simulink library "Displays_Lib"  (Simulink 6.6)
PostLoadFcn:
  | ,try, rti_mdl_postloadfcn(bdroot, 'UpdateModel', 260, 'rti1005'); catch, disp(lasterr); end,
undefined symbols (not defined in the file or in its folder): Timestep
libraries: Displays_Lib x5, udpbs x4, simulink x1
settings Model: Creator=W.J.Leath  LastModifiedBy=cbuttril  ExtModeAutoUpdateStatusClock=off

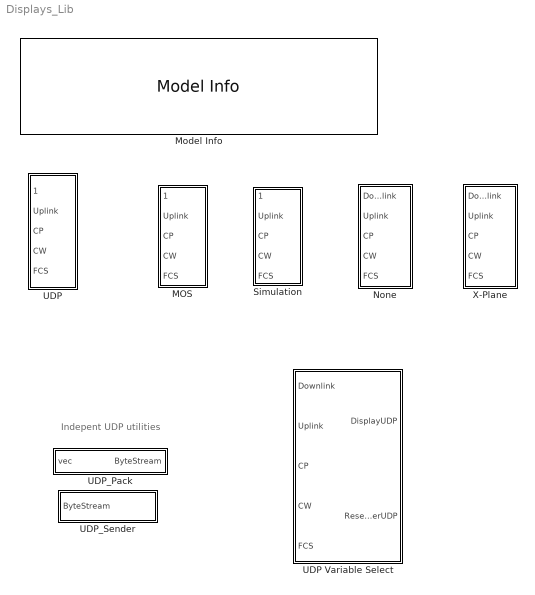
== system Displays_Lib ==
  note: Indepent UDP utilities
  MOS : Subsystem
  Model Info : simulink/Model-Wide Utilities/Model Info  SystemSampleTime=-1  InitialBlockCM=None  BlockCM=None  Frame=on  DisplayStringWithTags=|  HorizontalTextAlignment=Center  LeftAlignmentValue=0.5  SourceBlockDiagram=Displays_Lib  TagMaxNumber=20
      | Developed using Matlab Release 2007a
      | 
      | SVN:%<ModelVersion>
      | Modified: %<ModifiedDate>
  None : Subsystem
  Simulation : Subsystem
  UDP : Subsystem  BlockChoice=MOS
      settings: TemplateBlock=self  MemberBlocks=MOS,None,Simulation,X-Plane
  UDP Variable Select : Subsystem
  UDP_Pack : Subsystem  mask(UDPPacker){DataType=double, EndianListNdx=Little Endian (Intel)}
      mask prompts: DataType "Input datatype"; EndianListNdx "Native Byte Order"
      mask help: Takes vectors of doubles or uint32s and forms a packed bytestream suitable for sending via UDP.
      mask init:
      | IsBigEndian=boolean(EndianListNdx-1);
      | switch DataType
      |     case 'uint32'
      |         vbytes = 4;
      |     case 'double'
      |         vbytes = 8;
      | end
      mask StyleString: popup(uint32|double),popup(Little Endian (Intel)|Big Endian (dSpace))
      mask Display:
      | port_label('input',1,DataType)
      | port_label('output',1,'ByteStream')
  UDP_Sender : Subsystem  mask(UDP_Send){UDP_Port=5001}
      mask prompts: UDP_Port "UDP Port to Send Message to"
      mask help: Sends a uint8 bytesteam to the specified UDP port. Must be able to open a different port on local machine to estabilish the socket. By convention the local socket is opened one port below the destination port. For example, to send a message to port 5001, this block must be able to open a socket on port 5000 on the local machine.
  X-Plane : Subsystem

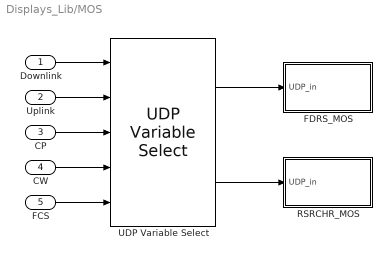
== system Displays_Lib/MOS ==
  Downlink : Inport
  Uplink : Inport  Port=2
  CP : Inport  Port=3
  CW : Inport  Port=4
  FCS : Inport  Port=5
  FDRS_MOS : Subsystem
  RSRCHR_MOS : Subsystem
  UDP Variable Select : Displays_Lib/UDP Variable Select  SystemSampleTime=-1
      link override UDP_Pack: EndianListNdx=Big Endian (dSpace)
      link override UDP_Pack0: EndianListNdx=Big Endian (dSpace)
      link override UDP_Pack1: EndianListNdx=Big Endian (dSpace)
      link override UDP_Pack2: EndianListNdx=Big Endian (dSpace)
      link override UDP_Pack3: EndianListNdx=Big Endian (dSpace)
  wires:
  Downlink/1 -> UDP Variable Select/1
  Uplink/1 -> UDP Variable Select/2
  CP/1 -> UDP Variable Select/3
  FCS/1 -> UDP Variable Select/5
  CW/1 -> UDP Variable Select/4
  UDP Variable Select/1 -> FDRS_MOS/1(UDP_in)
  UDP Variable Select/2 -> RSRCHR_MOS/1(UDP_in)

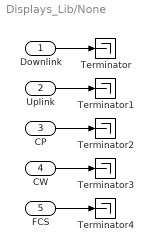
== system Displays_Lib/None ==
  Downlink : Inport
  Uplink : Inport  Port=2
  CP : Inport  Port=3
  CW : Inport  Port=4
  FCS : Inport  Port=5
  Terminator{,1..4} (5 alike) : Terminator
  wires:
  Downlink/1 -> Terminator/1
  Uplink/1 -> Terminator1/1
  CP/1 -> Terminator2/1
  CW/1 -> Terminator3/1
  FCS/1 -> Terminator4/1

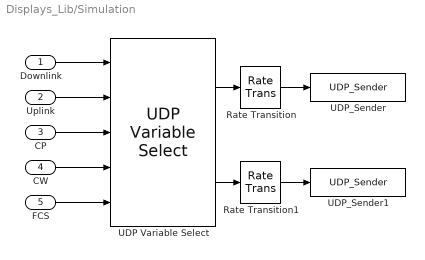
== system Displays_Lib/Simulation ==
  Downlink : Inport
  Uplink : Inport  Port=2
  CP : Inport  Port=3
  CW : Inport  Port=4
  FCS : Inport  Port=5
  Rate Transition : RateTransition  Deterministic=off  OutPortSampleTime=Timestep*4
  Rate Transition1 : RateTransition  Deterministic=off  OutPortSampleTime=Timestep*4
  UDP Variable Select : Displays_Lib/UDP Variable Select  SystemSampleTime=-1
  UDP_Sender : Displays_Lib/UDP_Sender  SystemSampleTime=-1  UDP_Port=5500
  UDP_Sender1 : Displays_Lib/UDP_Sender  SystemSampleTime=-1  UDP_Port=5700
  wires:
  Downlink/1 -> UDP Variable Select/1
  Uplink/1 -> UDP Variable Select/2
  CP/1 -> UDP Variable Select/3
  FCS/1 -> UDP Variable Select/5
  CW/1 -> UDP Variable Select/4
  UDP Variable Select/1 -> Rate Transition/1
  UDP Variable Select/2 -> Rate Transition1/1
  Rate Transition/1 -> UDP_Sender/1
  Rate Transition1/1 -> UDP_Sender1/1

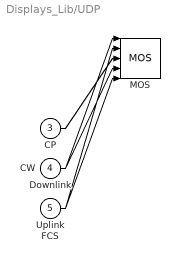
== system Displays_Lib/UDP ==
  Downlink : Inport
  Uplink : Inport  Port=2
  CP : Inport  Port=3
  CW : Inport  Port=4
  FCS : Inport  Port=5
  MOS : Displays_Lib/MOS  SystemSampleTime=-1
  wires:
  Downlink/1 -> MOS/1
  Uplink/1 -> MOS/2
  CP/1 -> MOS/3
  CW/1 -> MOS/4
  FCS/1 -> MOS/5

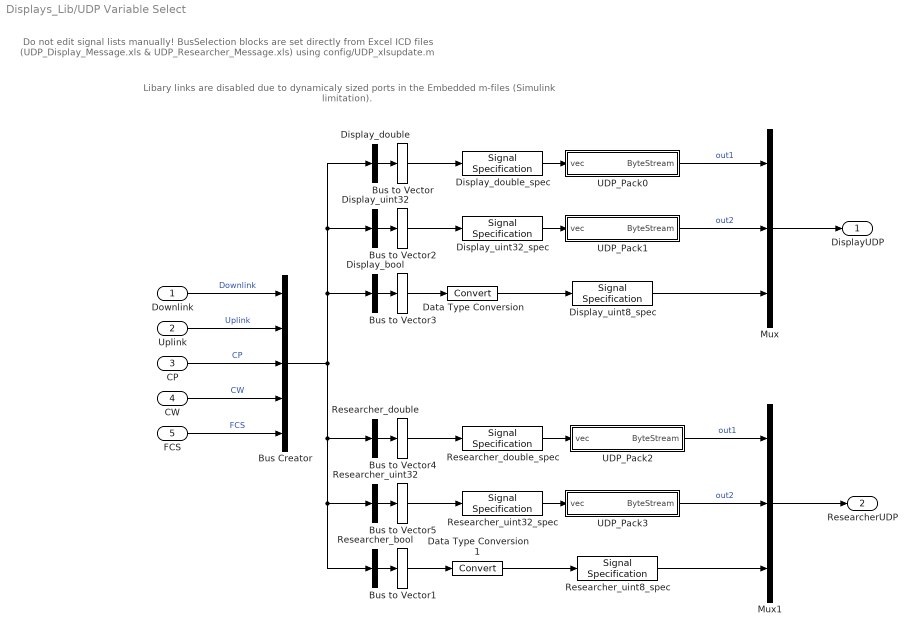
== system Displays_Lib/UDP Variable Select ==
  note: Libary links are disabled due to dynamicaly sized ports
      | in the Embedded m-files (Simulink limitation).
  note: Do not edit signal lists manually!  BusSelection blocks are set directly from Excel ICD files
      | (UDP_Display_Message.xls & UDP_Researcher_Message.xls) using config/UDP_xlsupdate.m
  Downlink : Inport
  Uplink : Inport  Port=2
  CP : Inport  Port=3
  CW : Inport  Port=4
  FCS : Inport  Port=5
  Bus Creator : BusCreator  Inputs=5
  Bus to Vector{,1..5} (6 alike) : BusToVector
  Data Type Conversion : DataTypeConversion  OutDataTypeMode=uint8
  Data Type Conversion1 : DataTypeConversion  OutDataTypeMode=uint8
  Display_bool : BusSelector  OutputSignals=FCS.RPraw.FTE_mark,FCS.RPraw.TD_mark,FCS.RPraw.ENG_mark,FCS.RPraw.RES_mark,FCS.SPInput.gear_cmd,FCS.SPInput.handoff_switch,FCS.RPInput.Fuel_Intg,CW.LinkInop  OutputAsBus=on
  Display_double : BusSelector  OutputSignals=CP.AirData.vc,CP.AirData.vt,CP.CGVanesAcc.gwest,CP.Display.cg_mac,CP.Display.vstall_est_disp,CP.Display.vc_disp,CP.Display.alpha_disp,CP.Display.beta_disp,CP.Display.baro_alt,CP.Display.nz_disp,CP.Display.vv_fpm_disp,CP.Display.mag_heading_disp,CP.Display.alt_gps_disp,CP.Display.BUSMON1_disp,CP.Display.BUSMON2_disp,CP.Display.BUSMON3_disp,CP.Display.BUSMON4_disp,CP.Display.CPTV_disp,CP.Display.BAROV_disp,CP.Display.MAG3V_disp,CP.Display.RSS_disp,CP.Display.DL_RSS_disp,CP.Engine_Fuel.fuel_rem,CP.Engine_Fuel.fuel_flow_l,CP.Engine_Fuel.fuel_flow_r,CP.Engine_Fuel.fuel_used,CP.Engine_Fuel.time_rem,CP.Engine_Fuel.rpm_left,CP.Engine_Fuel.rpm_right,CP.Engine_Fuel.rpml_ATcmd,CP.Engine_Fuel.rpmr_ATcmd,CP.Engine_Fuel.rpml_RPcmd,CP.Engine_Fuel.rpmr_RPcmd,CP.Engine_Fuel.rpml_SPcmd,CP.Engine_Fuel.rpmr_SPcmd,CP.Nav.vcdot,CP.Nav.vgnav,CP.Nav.windspd,CP.Nav.winddir,CP.Nav.gammav,CP.Nav.gndtrack,CP.Surfaces.RPele_cmd,CP.Surfaces.aildiff,CP.Surfaces.elevave,CP.Surfaces.rudave,CP.CP_constants.altimeter_setting,CP.Offset_Landing.baro_alt_HUD,CP.Offset_Landing.mag_heading_disp_HUD,CP.Offset_Landing.gndtrack_HUD,CP.Offset_Landing.psideg_HUD,CP.Offset_Landing.latdeg_HUD,CP.Offset_Landing.londeg_HUD,Downlink.ADC.EGTR,Downlink.ADC.EGTL,Downlink.ADC.SSCS,Downlink.ADC.PSL,Downlink.ADC.PDL,Downlink.ADC.PSR,Downlink.ADC.PDR,Downlink.ADC.AILL,Downlink.ADC.AILR,Downlink.ADC.ELLOB,Downlink.ADC.ELLIB,Downlink.ADC.ELROB,Downlink.ADC.ELRIB,Downlink.ADC.RUDU,Downlink.ADC.RUDL,Downlink.ADC.XACCEL,Downlink.ADC.YACCEL,Downlink.ADC.ZACCEL,Downlink.ADC.XGYRO,Downlink.ADC.YGYRO,Downlink.ADC.ZGYRO,Downlink.ADC.TEMPAMB,Downlink.Health.PacketErrorIndPort0,Downlink.Health.PacketErrorIndPort1,Downlink.Health.PacketErrorIndPort2,Downlink.Health.PacketErrorIndPort3,Downlink.MIDG.MSG_10.TimeStamp,Downlink.MIDG.MSG_10.pdeg,Downlink.MIDG.MSG_10.qdeg,Downlink.MIDG.MSG_10.rdeg,Downlink.MIDG.MSG_10.nxbody,Downlink.MIDG.MSG_10.nybody,Downlink.MIDG.MSG_10.nzbody,Downlink.MIDG.MSG_10.phideg,Downlink.MIDG.MSG_10.thetadeg,Downlink.MIDG.MSG_10.psideg,Downlink.MIDG.MSG_12.LAT_NAV,Downlink.MIDG.MSG_12.LON_NAV,Downlink.MIDG.MSG_1.MIDG_mode,FCS.AT.spd_cmd,FCS.Mode2.beta_cmd,FCS.Mode2.alpha_trim_cmd,FCS.Mode2.alpha_cmd,FCS.RPInput.throttle_L,FCS.RPInput.throttle_R,FCS.RPInput.lon_stk,FCS.RPInput.lat_stk,FCS.RPInput.pedal,FCS.RPInput.hat_lon,FCS.RPInput.hat_lat,FCS.RPInput.flap,FCS.RPInput.spd_brake,FCS.RPInput.Alpha_select,FCS.RPInput.Beta_select,FCS.RPInput.DynPress_select,FCS.RPInput.StatPress_select,FCS.Uplink_cmds.ELLOBC,FCS.Uplink_cmds.ELLIBC,FCS.Uplink_cmds.ELROBC,FCS.Uplink_cmds.ELRIBC,FCS.Uplink_cmds.AILLC,FCS.Uplink_cmds.SPLLOBC,FCS.Uplink_cmds.SPLLIBC,FCS.Uplink_cmds.SPLRIBC,FCS.Uplink_cmds.SPLROBC,FCS.Uplink_cmds.AILRC,FCS.Uplink_cmds.RUDUPC,FCS.Uplink_cmds.RUDLOC,FCS.Uplink_cmds.FLAPLOC,FCS.Uplink_cmds.FLAPLIC,FCS.Uplink_cmds.FLAPRIC,FCS.Uplink_cmds.FLAPROC,FCS.Uplink_cmds.GEARC,FCS.SPInput.throttle_cmd,FCS.SPInput.ail_cmd,FCS.SPInput.ele_cmd,FCS.SPInput.rud_cmd,FCS.SPInput.flap_cmd  OutputAsBus=on
  Display_double_spec : SignalSpecification  Dimensions=130  DataType=double
  Display_uint32 : BusSelector  OutputSignals=CW.warning_word,CW.caution_word,CW.advisory_word,FCS.FCS_Engage,FCS.FCS_Arm,FCS.Wavetrain.WT_status.WT_profile,FCS.Mode3.rFCL_select,FCS.MTF.MTF_profile,CW.StallTone  OutputAsBus=on
  Display_uint32_spec : SignalSpecification  Dimensions=9  DataType=uint32
  Display_uint8_spec : SignalSpecification  Dimensions=8  DataType=uint8
  Mux : Mux  Inputs=3
  Mux1 : Mux  Inputs=3
  Researcher_bool : BusSelector  OutputSignals=FCS.RPraw.gear  OutputAsBus=on
  Researcher_double : BusSelector  OutputSignals=Downlink.ADC.ALPHAVL,Downlink.ADC.BETAVL,Downlink.ADC.ALPHAVR,Downlink.ADC.BETAVR,Downlink.ADC.PSL,Downlink.ADC.PDL,Downlink.ADC.PSR,Downlink.ADC.PDR,Downlink.ADC.XACCEL,Downlink.ADC.YACCEL,Downlink.ADC.ZACCEL,Downlink.ADC.XGYRO,Downlink.ADC.YGYRO,Downlink.ADC.ZGYRO,Downlink.ADC.XMAG,Downlink.ADC.YMAG,Downlink.ADC.ZMAG,Downlink.ADC.XGYROT,Downlink.ADC.AILL,Downlink.ADC.AILR,Downlink.ADC.ELLOB,Downlink.ADC.ELLIB,Downlink.ADC.ELROB,Downlink.ADC.ELRIB,Downlink.ADC.RUDU,Downlink.ADC.RUDL,Downlink.ADC.FLAPLOB,Downlink.ADC.FLAPLIB,Downlink.ADC.FLAPRIB,Downlink.ADC.FLAPROB,Downlink.ADC.TEMPAMB,Downlink.ADC.RPML,Downlink.ADC.RPMR,Downlink.MIDG.MSG_10.TimeStamp,Downlink.MIDG.MSG_10.pdeg,Downlink.MIDG.MSG_10.qdeg,Downlink.MIDG.MSG_10.rdeg,Downlink.MIDG.MSG_10.nxbody,Downlink.MIDG.MSG_10.nybody,Downlink.MIDG.MSG_10.nzbody,Downlink.MIDG.MSG_10.phideg,Downlink.MIDG.MSG_10.thetadeg,Downlink.MIDG.MSG_10.psideg,Downlink.MIDG.MSG_10.QW,Downlink.MIDG.MSG_10.QX,Downlink.MIDG.MSG_10.QY,Downlink.MIDG.MSG_10.QZ,Downlink.MIDG.MSG_12.LAT_NAV,Downlink.MIDG.MSG_12.LON_NAV,Downlink.MIDG.MSG_12.HELIP_NAV,Downlink.MIDG.MSG_12.VEE_NAV,Downlink.MIDG.MSG_12.VN_NAV,Downlink.MIDG.MSG_12.VH_NAV,Uplink.AILLC,Uplink.AILRC,Uplink.ELLOBC,Uplink.ELLIBC,Uplink.ELROBC,Uplink.ELRIBC,Uplink.RUDUPC,Uplink.RUDLOC,Uplink.FLAPLIC,Uplink.FLAPLOC,Uplink.FLAPRIC,Uplink.FLAPROC,Uplink.THROTLC,Uplink.THROTRC,Uplink.GEARC,Uplink.SPLLIBC,Uplink.SPLLOBC,Uplink.SPLRIBC,Uplink.SPLROBC,CP.CGVanesAcc.gwest,CP.CGVanesAcc.cgx,CP.CGVanesAcc.cgy,CP.CGVanesAcc.cgz,CP.CGVanesAcc.ixx,CP.CGVanesAcc.iyy,CP.CGVanesAcc.izz,CP.CGVanesAcc.ixz,CP.CGVanesAcc.MIDG_nxcorr,CP.CGVanesAcc.MIDG_nycorr,CP.CGVanesAcc.MIDG_nzcorr,CP.CGVanesAcc.nxcorr,CP.CGVanesAcc.nycorr,CP.CGVanesAcc.nzcorr,CP.CGVanesAcc.alpha_l,CP.CGVanesAcc.beta_l,CP.CGVanesAcc.alpha_r,CP.CGVanesAcc.beta_r,CP.AirData.vt,CP.AirData.hpic,CP.Nav.windspd,CP.Nav.winddir,CP.Engine_Fuel.fuel_used,CP.Engine_Fuel.rpm_left,CP.Engine_Fuel.rpm_right,CP.Surfaces.aildiff,CP.Surfaces.elevave,CP.Surfaces.rudave,FCS.RPraw.throttle_L,FCS.RPraw.throttle_R,FCS.RPraw.lon_stk,FCS.RPraw.lat_stk,FCS.RPraw.pedal,FCS.RPraw.hat_lon,FCS.RPraw.hat_lat,FCS.RPraw.flap,FCS.RPraw.spd_brake,FCS.AT.spd_cmd,FCS.Mode2.beta_cmd,FCS.Mode2.alpha_trim_cmd,FCS.Mode2.alpha_cmd,FCS.Wavetrain.WT_cmds.dAILLC,FCS.Wavetrain.WT_cmds.dAILRC,FCS.Wavetrain.WT_cmds.dELLOBC,FCS.Wavetrain.WT_cmds.dELLIBC,FCS.Wavetrain.WT_cmds.dELROBC,FCS.Wavetrain.WT_cmds.dELRIBC,FCS.Wavetrain.WT_cmds.dRUDUPC,FCS.Wavetrain.WT_cmds.dRUDLOC,FCS.Wavetrain.WT_cmds.dFLAPLIC,FCS.Wavetrain.WT_cmds.dFLAPLOC,FCS.Wavetrain.WT_cmds.dFLAPRIC,FCS.Wavetrain.WT_cmds.dFLAPROC,FCS.Wavetrain.WT_cmds.dTHROTLC,FCS.Wavetrain.WT_cmds.dTHROTRC,FCS.Wavetrain.WT_cmds.dSPLLIBC,FCS.Wavetrain.WT_cmds.dSPLLOBC,FCS.Wavetrain.WT_cmds.dSPLRIBC,FCS.Wavetrain.WT_cmds.dSPLROBC,FCS.Mode3.UserData.UserData1,FCS.Mode3.UserData.UserData2,FCS.Mode3.UserData.UserData3,FCS.Mode3.UserData.UserData4,FCS.Mode3.UserData.UserData5,FCS.Mode3.UserData.UserData6,FCS.Mode3.UserData.UserData7,FCS.Mode3.UserData.UserData8,FCS.Mode3.UserData.UserData9,FCS.Mode3.UserData.UserData10,FCS.Mode3.UserData.UserData11,FCS.Mode3.UserData.UserData12,FCS.Mode3.UserData.UserData13,FCS.Mode3.UserData.UserData14,FCS.Mode3.UserData.UserData15,FCS.Mode3.UserData.UserData16,FCS.Mode3.UserData.UserData17,FCS.Mode3.UserData.UserData18,FCS.Mode3.UserData.UserData19,FCS.Mode3.UserData.UserData20,FCS.Mode3.UserData.UserData21,FCS.Mode3.UserData.UserData22,FCS.Mode3.UserData.UserData23,FCS.Mode3.UserData.UserData24,FCS.Mode3.UserData.UserData25,FCS.Mode3.UserData.UserData26,FCS.Mode3.UserData.UserData27,FCS.Mode3.UserData.UserData28,FCS.Mode3.UserData.UserData29,FCS.Mode3.UserData.UserData30  OutputAsBus=on
  Researcher_double_spec : SignalSpecification  Dimensions=161  DataType=double
  Researcher_uint32 : BusSelector  OutputSignals=FCS.FCS_Engage,FCS.FCS_Arm,FCS.Mode3.rFCL_select,FCS.MTF.MTF_profile,FCS.Wavetrain.WT_status.WT_profile  OutputAsBus=on
  Researcher_uint32_spec : SignalSpecification  Dimensions=5  DataType=uint32
  Researcher_uint8_spec : SignalSpecification  Dimensions=1  DataType=uint8
  UDP_Pack0 : Subsystem  AncestorBlock=Displays_Lib/UDP_Pack  mask(UDPPacker){DataType=double, EndianListNdx=Little Endian (Intel)}
      mask prompts: DataType "Input datatype"; EndianListNdx "Native Byte Order"
      mask help: Takes vectors of doubles or uint32s and forms a packed bytestream suitable for sending via UDP.
      mask init:
      | IsBigEndian=boolean(EndianListNdx-1);
      | switch DataType
      |     case 'uint32'
      |         vbytes = 4;
      |     case 'double'
      |         vbytes = 8;
      | end
      mask StyleString: popup(uint32|double),popup(Little Endian (Intel)|Big Endian (dSpace))
      mask Display:
      | port_label('input',1,DataType)
      | port_label('output',1,'ByteStream')
  UDP_Pack1 : Subsystem  AncestorBlock=Displays_Lib/UDP_Pack  mask(UDPPacker){DataType=uint32, EndianListNdx=Little Endian (Intel)}
      mask prompts: DataType "Input datatype"; EndianListNdx "Native Byte Order"
      mask help: Takes vectors of doubles or uint32s and forms a packed bytestream suitable for sending via UDP.
      mask init:
      | IsBigEndian=boolean(EndianListNdx-1);
      | switch DataType
      |     case 'uint32'
      |         vbytes = 4;
      |     case 'double'
      |         vbytes = 8;
      | end
      mask StyleString: popup(uint32|double),popup(Little Endian (Intel)|Big Endian (dSpace))
      mask Display:
      | port_label('input',1,DataType)
      | port_label('output',1,'ByteStream')
  UDP_Pack2 : Subsystem  AncestorBlock=Displays_Lib/UDP_Pack  mask(UDPPacker){DataType=double, EndianListNdx=Little Endian (Intel)}
      mask prompts: DataType "Input datatype"; EndianListNdx "Native Byte Order"
      mask help: Takes vectors of doubles or uint32s and forms a packed bytestream suitable for sending via UDP.
      mask init:
      | IsBigEndian=boolean(EndianListNdx-1);
      | switch DataType
      |     case 'uint32'
      |         vbytes = 4;
      |     case 'double'
      |         vbytes = 8;
      | end
      mask StyleString: popup(uint32|double),popup(Little Endian (Intel)|Big Endian (dSpace))
      mask Display:
      | port_label('input',1,DataType)
      | port_label('output',1,'ByteStream')
  UDP_Pack3 : Subsystem  AncestorBlock=Displays_Lib/UDP_Pack  mask(UDPPacker){DataType=uint32, EndianListNdx=Little Endian (Intel)}
      mask prompts: DataType "Input datatype"; EndianListNdx "Native Byte Order"
      mask help: Takes vectors of doubles or uint32s and forms a packed bytestream suitable for sending via UDP.
      mask init:
      | IsBigEndian=boolean(EndianListNdx-1);
      | switch DataType
      |     case 'uint32'
      |         vbytes = 4;
      |     case 'double'
      |         vbytes = 8;
      | end
      mask StyleString: popup(uint32|double),popup(Little Endian (Intel)|Big Endian (dSpace))
      mask Display:
      | port_label('input',1,DataType)
      | port_label('output',1,'ByteStream')
  DisplayUDP : Outport
  ResearcherUDP : Outport  Port=2
  wires:
  UDP_Pack0/1(ByteStream) -> Mux/1  "out1"
  UDP_Pack1/1(ByteStream) -> Mux/2  "out2"
  Display_uint32_spec/1 -> UDP_Pack1/1(vec)
  Display_uint8_spec/1 -> Mux/3
  Researcher_double_spec/1 -> UDP_Pack2/1(vec)
  Downlink/1 -> Bus Creator/1  "Downlink"
  Uplink/1 -> Bus Creator/2  "Uplink"
  CP/1 -> Bus Creator/3  "CP"
  CW/1 -> Bus Creator/4  "CW"
  FCS/1 -> Bus Creator/5  "FCS"
  Bus Creator/1 -> Display_bool/1, Researcher_double/1, Researcher_uint32/1, Researcher_bool/1, Display_double/1, Display_uint32/1
  Researcher_double/1 -> Bus to Vector4/1
  Display_bool/1 -> Bus to Vector3/1
  Display_uint32/1 -> Bus to Vector2/1
  Display_double/1 -> Bus to Vector/1
  Researcher_uint32_spec/1 -> UDP_Pack3/1(vec)
  Researcher_uint32/1 -> Bus to Vector5/1
  UDP_Pack2/1(ByteStream) -> Mux1/1  "out1"
  UDP_Pack3/1(ByteStream) -> Mux1/2  "out2"
  Mux1/1 -> ResearcherUDP/1
  Mux/1 -> DisplayUDP/1
  Bus to Vector2/1 -> Display_uint32_spec/1
  Bus to Vector3/1 -> Data Type Conversion/1
  Bus to Vector4/1 -> Researcher_double_spec/1
  Bus to Vector5/1 -> Researcher_uint32_spec/1
  Researcher_bool/1 -> Bus to Vector1/1
  Bus to Vector1/1 -> Data Type Conversion1/1
  Researcher_uint8_spec/1 -> Mux1/3
  Data Type Conversion/1 -> Display_uint8_spec/1
  Data Type Conversion1/1 -> Researcher_uint8_spec/1
  Display_double_spec/1 -> UDP_Pack0/1(vec)
  Bus to Vector/1 -> Display_double_spec/1

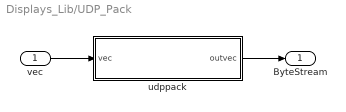
== system Displays_Lib/UDP_Pack ==
  vec : Inport
  udppack : Stateflow chart
  ByteStream : Outport
  wires:
  udppack/1(outvec) -> ByteStream/1
  vec/1 -> udppack/1(vec)

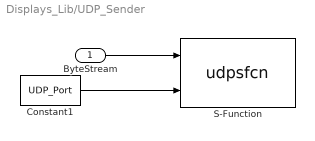
== system Displays_Lib/UDP_Sender ==
  ByteStream : Inport
  Constant1 : Constant  Value=UDP_Port  OutDataTypeMode=uint32
  S-Function : S-Function  FunctionName=udpsfcn
  wires:
  Constant1/1 -> S-Function/2
  ByteStream/1 -> S-Function/1

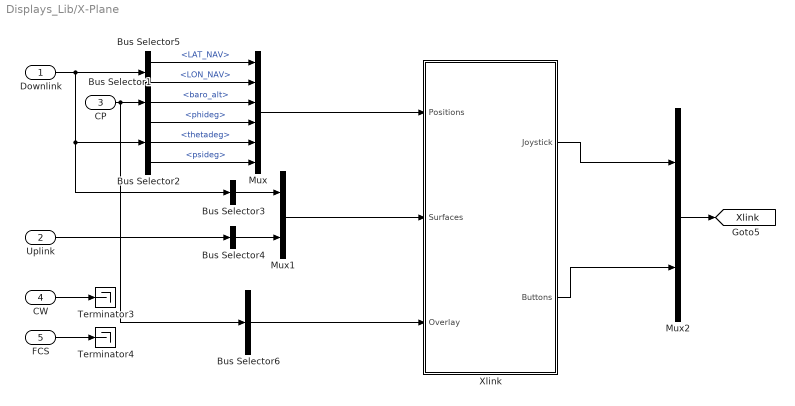
== system Displays_Lib/X-Plane ==
  Downlink : Inport
  Uplink : Inport  Port=2
  CP : Inport  Port=3
  CW : Inport  Port=4
  FCS : Inport  Port=5
  Bus Selector1 : BusSelector  OutputSignals=Display.baro_alt
  Bus Selector2 : BusSelector  OutputSignals=MIDG.MSG_10.phideg,MIDG.MSG_10.thetadeg,MIDG.MSG_10.psideg
  Bus Selector3 : BusSelector  OutputSignals=ADC.AILL,ADC.ELLOB,ADC.RUDU,ADC.FLAPROB  OutputAsBus=on
  Bus Selector4 : BusSelector  OutputSignals=SPLLOBC,GEARC  OutputAsBus=on
  Bus Selector5 : BusSelector  OutputSignals=MIDG.MSG_12.LAT_NAV,MIDG.MSG_12.LON_NAV
  Bus Selector6 : BusSelector  OutputSignals=CGVanesAcc.alpha,CGVanesAcc.beta,AirData.vc  OutputAsBus=on
  Mux : Mux  Inputs=6
  Mux1 : Mux  Inputs=2
  Mux2 : Mux  Inputs=2
  Terminator3 : Terminator
  Terminator4 : Terminator
  Xlink : Subsystem  mask(Xlink){HUDCell={'alpha','beta','Velocity'}}
      mask prompts: HUDCell "Lables for HUD, (cell array)"
      mask help:
      | Input Positions and Surfaces for X-Plane Visualization.
      |   Positions - [ Latitude, Longitude, Altitude, Roll, Pitch, Yaw] % degrees and ft.
      |   Surfaces  - [ Aileron, Elevator, Rudder, Flaps, Spoiler, GearDown] % deg and 0/1
      |
      | Output is Joysick axes and Button pushes.
      |   Joystick - First 16 axes
      |   Buttons  - 16 buttons as assigned to Xlink in X-Plane
      mask init:
      | if isempty(HUDCell) HUDCell=cell(6,1); end
      | HUDTextArray = uint8(zeros(90,1));
      | 
      | % loop through names, assign to string arrays
      | for i=1:min(length(HUDCell),6);
      |   if length(HUDCell{i})>14 HUDCell{i}=HUDCell{i}(1:14); end
      |   if length(HUDCell{i}>0),
      |     HUDTextArray((i-1)*15+1:(i-1)*15+length(HUDCell{i})) = uint8(HUDCell{i});
      |   end
      | end
  tag scope: Xlink=global
  wires:
  Bus Selector6/1 -> Xlink/3(Overlay)
  Xlink/2(Buttons) -> Mux2/2
  Downlink/1 -> Bus Selector3/1, Bus Selector2/1, Bus Selector5/1
  CW/1 -> Terminator3/1
  FCS/1 -> Terminator4/1
  Bus Selector2/1 -> Mux/4  "<phideg>"
  Bus Selector2/2 -> Mux/5  "<thetadeg>"
  CP/1 -> Bus Selector6/1, Bus Selector1/1
  Uplink/1 -> Bus Selector4/1
  Bus Selector3/1 -> Mux1/1
  Mux1/1 -> Xlink/2(Surfaces)
  Bus Selector2/3 -> Mux/6  "<psideg>"
  Bus Selector1/1 -> Mux/3  "<baro_alt>"
  Bus Selector5/1 -> Mux/1  "<LAT_NAV>"
  Bus Selector5/2 -> Mux/2  "<LON_NAV>"
  Xlink/1(Joystick) -> Mux2/1
  Mux2/1 -> [Xlink]
  Bus Selector4/1 -> Mux1/2
  Mux/1 -> Xlink/1(Positions)

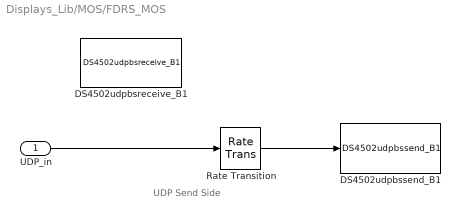
== system Displays_Lib/MOS/FDRS_MOS ==
  note: UDP Send Side
  UDP_in : Inport
  DS4502udpbsreceive_B1 : udpbs/DS4502udpbsreceive_B1  SystemSampleTime=-1  BoardNo=1  LocalIp10=192.168.1.155  LocalIp11=1  LocalIp12=1  LocalIp13=1  SourceIp20=0.0.0.0  SourceIp21=1  SourceIp22=1  SourceIp23=1  Port=5500  Timeout=0  Sample_time=-1  Overflow_Flush=off  LocalIp=1  SourceIp=1  DSProperties=struct('RTI',struct('Version',uint32(3),'BlockType',struct('isSLSource',logical(0),'isSLSink',logical(0),'isHWSource',logical(0),'isHWSink',logical(0),'isSetup',logical(0),'isInline',logical(0),'isNonInline',logical(1),'isInterrupt',logical(0),'isChannelwise',logical(0)),'Identifier','udpbsreceive','IOBoardType','DS4502','UnitType','UDP','BlockSet','UDPBS','DialogType','SL','SlaveProcessor','NONE'))  RTIBlockInterface=struct('OutputPortsActive',0,'OutputPortsWidth',int32(0),'MaskDescription',['Receives UDP-based datagrams for a connected socket and stores these data in the port buffer within the corresponding port memory structure.'],'BlockDisplay',{{['UDP Receive'],'middle'}},'IconTransparency','on','BlockName',struct('Token',{{'DS4502udpbsreceive_B'}},'BlockParam',{{'BoardNo'}}),'InitLevel',3)  RTIBlockParameters=struct('BoardNo',{{1,'ON',[1 16]}},'LocalIp10',{{'192.168.1.155','OFF',[]}},'LocalIp11',{{'1','OFF',[]}},'LocalIp12',{{'1','OFF',[]}},'LocalIp13',{{'1','OFF',[]}},'SourceIp20',{{'0.0.0.0','OFF',[]}},'SourceIp21',{{'1','OFF',[]}},'SourceIp22',{{'1','OFF',[]}},'SourceIp23',{{'1','OFF',[]}},'Port',{{5500,'ON',[1025 65535]}},'Timeout',{{0,'ON',[0 1]}},'Sample_time',{{-1,'OFF',[]}},'Overflow_Flush',{{logical(0),'OFF',[]}},'LocalIp',{{'1','OFF',[]}},'SourceIp',{{'1','OFF',[]}})  RTISFcnParameters=struct('BoardNo','double','LocalIp10','char','LocalIp11','double','LocalIp12','double','LocalIp13','double','SourceIp20','char','SourceIp21','double','SourceIp22','double','SourceIp23','double','Port','double','Timeout','double','Sample_time','double','Overflow_Flush','double','LocalIp','char','SourceIp','char')  RTIBlockParaDefault=struct('BoardNo',1,'LocalIp10','192.168.100.1','LocalIp11','1','LocalIp12','1','LocalIp13','1','SourceIp20','192.168.100.2','SourceIp21','1','SourceIp22','1','SourceIp23','1','Port',5000,'Timeout',0.00022,'Sample_time',-1,'Overflow_Flush',0,'LocalIp','1','SourceIp','1')
  DS4502udpbssend_B1 : udpbs/DS4502udpbssend_B1  SystemSampleTime=-1  BoardNo=1  LocalIp10=192.168.1.155  LocalIp11=1  LocalIp12=1  LocalIp13=1  DestinationIp20=255.255.255.255  DestinationIp21=1  DestinationIp22=1  DestinationIp23=1  Port=5500  Timeout=1/250  sample_time=-1  LocalIp=1  DestinationIp=1  DSProperties=struct('RTI',struct('Version',uint32(3),'BlockType',struct('isSLSource',logical(0),'isSLSink',logical(1),'isHWSource',logical(0),'isHWSink',logical(1),'isSetup',logical(0),'isInline',logical(0),'isNonInline',logical(1),'isInterrupt',logical(0),'isChannelwise',logical(0)),'DialogType','SL','Identifier','udpbssend','IOBoardType','DS4502','UnitType','UDP','BlockSet','UDPBS','SlaveProcessor','NONE'))  RTIBlockInterface=struct('MaskDescription',['Sends UDP-based datagrams for a connected socket to an Ethernet communication partner.'],'InputPortsActive',1,'InputPortsWidth',{{'DYNAMICALLY_SIZED'}},'InputPortsDataType',{{'SS_DOUBLE'}},'InputPortsName',{{'In'}},'BlockDisplay',{{['UDP Send'],'middle'}},'IconTransparency','on','BlockName',struct('Token',{{'DS4502udpbssend_B'}},'BlockParam',{{'BoardNo'}}),'InitLevel',3)  RTIBlockParameters=struct('BoardNo',{{1,'ON',[1 16]}},'LocalIp10',{{'192.168.1.155','OFF',[]}},'LocalIp11',{{'1','OFF',[]}},'LocalIp12',{{'1','OFF',[]}},'LocalIp13',{{'1','OFF',[]}},'DestinationIp20',{{'255.255.255.255','OFF',[]}},'DestinationIp21',{{'1','OFF',[]}},'DestinationIp22',{{'1','OFF',[]}},'DestinationIp23',{{'1','OFF',[]}},'Port',{{5500,'ON',[1025 65535]}},'Timeout',{{0.004,'ON',[0 1]}},'sample_time',{{-1,'OFF',[]}},'LocalIp',{{'1','OFF',[]}},'DestinationIp',{{'1','OFF',[]}})  RTISFcnParameters=struct('BoardNo','double','LocalIp10','char','LocalIp11','double','LocalIp12','double','LocalIp13','double','DestinationIp20','char','DestinationIp21','double','DestinationIp22','double','DestinationIp23','double','Port','double','Timeout','double','sample_time','double','LocalIp','char','DestinationIp','char')  RTIBlockParaDefault=struct('BoardNo',1,'LocalIp10','192.168.100.1','LocalIp11','1','LocalIp12','1','LocalIp13','1','DestinationIp20','192.168.100.2','DestinationIp21','1','DestinationIp22','1','DestinationIp23','1','Port',5000,'Timeout',0.00022,'sample_time',-1,'LocalIp','1','DestinationIp','1')
  Rate Transition : RateTransition  Deterministic=off  OutPortSampleTime="[Timestep*10.0  0.0]"
  wires:
  UDP_in/1 -> Rate Transition/1
  Rate Transition/1 -> DS4502udpbssend_B1/1

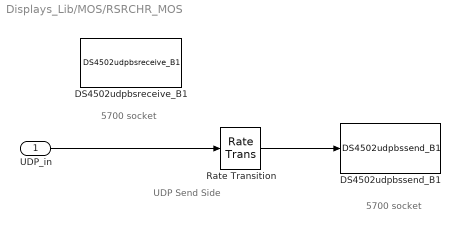
== system Displays_Lib/MOS/RSRCHR_MOS ==
  note: 5700 socket
  note: 5700 socket
  note: UDP Send Side
  UDP_in : Inport
  DS4502udpbsreceive_B1 : udpbs/DS4502udpbsreceive_B1  SystemSampleTime=-1  BoardNo=1  LocalIp10=192.168.1.155  LocalIp11=1  LocalIp12=1  LocalIp13=1  SourceIp20=0.0.0.0  SourceIp21=1  SourceIp22=1  SourceIp23=1  Port=5700  Timeout=0  Sample_time=-1  Overflow_Flush=off  LocalIp=1  SourceIp=1  DSProperties=struct('RTI',struct('Version',uint32(3),'BlockType',struct('isSLSource',logical(0),'isSLSink',logical(0),'isHWSource',logical(0),'isHWSink',logical(0),'isSetup',logical(0),'isInline',logical(0),'isNonInline',logical(1),'isInterrupt',logical(0),'isChannelwise',logical(0)),'Identifier','udpbsreceive','IOBoardType','DS4502','UnitType','UDP','BlockSet','UDPBS','DialogType','SL','SlaveProcessor','NONE'))  RTIBlockInterface=struct('OutputPortsActive',0,'OutputPortsWidth',int32(0),'MaskDescription',['Receives UDP-based datagrams for a connected socket and stores these data in the port buffer within the corresponding port memory structure.'],'BlockDisplay',{{['UDP Receive'],'middle'}},'IconTransparency','on','BlockName',struct('Token',{{'DS4502udpbsreceive_B'}},'BlockParam',{{'BoardNo'}}),'InitLevel',3)  RTIBlockParameters=struct('BoardNo',{{1,'ON',[1 16]}},'LocalIp10',{{'192.168.1.155','OFF',[]}},'LocalIp11',{{'1','OFF',[]}},'LocalIp12',{{'1','OFF',[]}},'LocalIp13',{{'1','OFF',[]}},'SourceIp20',{{'0.0.0.0','OFF',[]}},'SourceIp21',{{'1','OFF',[]}},'SourceIp22',{{'1','OFF',[]}},'SourceIp23',{{'1','OFF',[]}},'Port',{{5700,'ON',[1025 65535]}},'Timeout',{{0,'ON',[0 1]}},'Sample_time',{{-1,'OFF',[]}},'Overflow_Flush',{{logical(0),'OFF',[]}},'LocalIp',{{'1','OFF',[]}},'SourceIp',{{'1','OFF',[]}})  RTISFcnParameters=struct('BoardNo','double','LocalIp10','char','LocalIp11','double','LocalIp12','double','LocalIp13','double','SourceIp20','char','SourceIp21','double','SourceIp22','double','SourceIp23','double','Port','double','Timeout','double','Sample_time','double','Overflow_Flush','double','LocalIp','char','SourceIp','char')  RTIBlockParaDefault=struct('BoardNo',1,'LocalIp10','192.168.100.1','LocalIp11','1','LocalIp12','1','LocalIp13','1','SourceIp20','192.168.100.2','SourceIp21','1','SourceIp22','1','SourceIp23','1','Port',5000,'Timeout',0.00022,'Sample_time',-1,'Overflow_Flush',0,'LocalIp','1','SourceIp','1')
  DS4502udpbssend_B1 : udpbs/DS4502udpbssend_B1  SystemSampleTime=-1  BoardNo=1  LocalIp10=192.168.1.155  LocalIp11=1  LocalIp12=1  LocalIp13=1  DestinationIp20=255.255.255.255  DestinationIp21=1  DestinationIp22=1  DestinationIp23=1  Port=5700  Timeout=1/250  sample_time=-1  LocalIp=1  DestinationIp=1  DSProperties=struct('RTI',struct('Version',uint32(3),'BlockType',struct('isSLSource',logical(0),'isSLSink',logical(1),'isHWSource',logical(0),'isHWSink',logical(1),'isSetup',logical(0),'isInline',logical(0),'isNonInline',logical(1),'isInterrupt',logical(0),'isChannelwise',logical(0)),'DialogType','SL','Identifier','udpbssend','IOBoardType','DS4502','UnitType','UDP','BlockSet','UDPBS','SlaveProcessor','NONE'))  RTIBlockInterface=struct('MaskDescription',['Sends UDP-based datagrams for a connected socket to an Ethernet communication partner.'],'InputPortsActive',1,'InputPortsWidth',{{'DYNAMICALLY_SIZED'}},'InputPortsDataType',{{'SS_DOUBLE'}},'InputPortsName',{{'In'}},'BlockDisplay',{{['UDP Send'],'middle'}},'IconTransparency','on','BlockName',struct('Token',{{'DS4502udpbssend_B'}},'BlockParam',{{'BoardNo'}}),'InitLevel',3)  RTIBlockParameters=struct('BoardNo',{{1,'ON',[1 16]}},'LocalIp10',{{'192.168.1.155','OFF',[]}},'LocalIp11',{{'1','OFF',[]}},'LocalIp12',{{'1','OFF',[]}},'LocalIp13',{{'1','OFF',[]}},'DestinationIp20',{{'255.255.255.255','OFF',[]}},'DestinationIp21',{{'1','OFF',[]}},'DestinationIp22',{{'1','OFF',[]}},'DestinationIp23',{{'1','OFF',[]}},'Port',{{5700,'ON',[1025 65535]}},'Timeout',{{0.004,'ON',[0 1]}},'sample_time',{{-1,'OFF',[]}},'LocalIp',{{'1','OFF',[]}},'DestinationIp',{{'1','OFF',[]}})  RTISFcnParameters=struct('BoardNo','double','LocalIp10','char','LocalIp11','double','LocalIp12','double','LocalIp13','double','DestinationIp20','char','DestinationIp21','double','DestinationIp22','double','DestinationIp23','double','Port','double','Timeout','double','sample_time','double','LocalIp','char','DestinationIp','char')  RTIBlockParaDefault=struct('BoardNo',1,'LocalIp10','192.168.100.1','LocalIp11','1','LocalIp12','1','LocalIp13','1','DestinationIp20','192.168.100.2','DestinationIp21','1','DestinationIp22','1','DestinationIp23','1','Port',5000,'Timeout',0.00022,'sample_time',-1,'LocalIp','1','DestinationIp','1')
  Rate Transition : RateTransition  Deterministic=off  OutPortSampleTime="[Timestep*10.0  Timestep*3.0]"
  wires:
  Rate Transition/1 -> DS4502udpbssend_B1/1
  UDP_in/1 -> Rate Transition/1

== system Displays_Lib/UDP Variable Select/UDP_Pack0 ==
  vec : Inport
  udppack : Stateflow chart
  ByteStream : Outport
  wires:
  vec/1 -> udppack/1(vec)
  udppack/1(outvec) -> ByteStream/1

== system Displays_Lib/UDP Variable Select/UDP_Pack1 ==
  vec : Inport
  udppack : Stateflow chart
  ByteStream : Outport
  wires:
  vec/1 -> udppack/1(vec)
  udppack/1(outvec) -> ByteStream/1

== system Displays_Lib/UDP Variable Select/UDP_Pack2 ==
  vec : Inport
  udppack : Stateflow chart
  ByteStream : Outport
  wires:
  vec/1 -> udppack/1(vec)
  udppack/1(outvec) -> ByteStream/1

== system Displays_Lib/UDP Variable Select/UDP_Pack3 ==
  vec : Inport
  udppack : Stateflow chart
  ByteStream : Outport
  wires:
  vec/1 -> udppack/1(vec)
  udppack/1(outvec) -> ByteStream/1

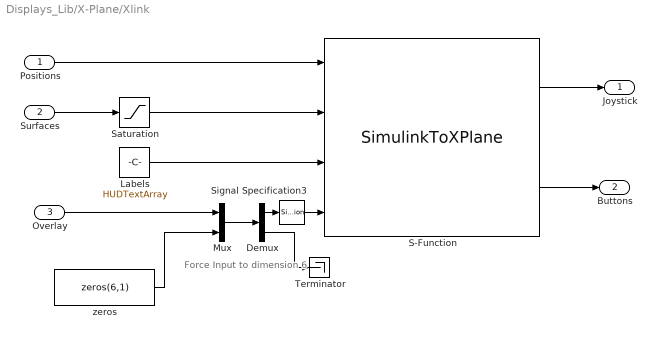
== system Displays_Lib/X-Plane/Xlink ==
  note: Force Input to
      | dimension 6
  Positions : Inport
  Surfaces : Inport  Port=2
  Overlay : Inport  Port=3
  Demux : Demux  Outputs=[6 -1]
  Labels : Constant  Value=HUDTextArray  OutDataTypeMode=uint8
  Mux : Mux  Inputs=2
  S-Function : S-Function  FunctionName=SimulinkToXPlane
  Saturation : Saturate  UpperLimit=[180*ones(5,1); 1]  LowerLimit=[-180*ones(5,1); 0]
  Signal Specification3 : SignalSpecification  Dimensions=6
  Terminator : Terminator
  zeros : Constant  Value=zeros(6,1)  OutDataTypeMode=double
  Joystick : Outport
  Buttons : Outport  Port=2
  wires:
  Demux/2 -> Terminator/1
  Demux/1 -> Signal Specification3/1
  Mux/1 -> Demux/1
  zeros/1 -> Mux/2
  Overlay/1 -> Mux/1
  Labels/1 -> S-Function/3
  Saturation/1 -> S-Function/2
  S-Function/2 -> Buttons/1
  Surfaces/1 -> Saturation/1
  S-Function/1 -> Joystick/1
  Positions/1 -> S-Function/1
  Signal Specification3/1 -> S-Function/4

== matlab function UDP Variable Select/UDP_Pack0/udppack ==
  data: vec input double; vbytes parameter double; outvec output uint8; IsBigEndian parameter boolean
function outvec = udppack(vec,vbytes,IsBigEndian)
Nv = length(vec); % get sizes of input vectors
outvec=uint8(zeros(Nv*vbytes,1)); % Set output size

if ~IsBigEndian  % Little Endian: typecast, reshape to column-wise, flip, reshape to vector
    cvec = reshape(flipud(reshape(typecast(vec(:),'uint8'),vbytes,Nv)),Nv*vbytes,1);
else   % Big Endian: typecast
    cvec = typecast(vec(:),'uint8');
end

% (:) selector retains size of "outvec"
outvec(:) = cvec;

== matlab function UDP Variable Select/UDP_Pack1/udppack ==
  data: vec input double; vbytes parameter double; outvec output uint8; IsBigEndian parameter boolean
function outvec = udppack(vec,vbytes,IsBigEndian)
Nv = length(vec); % get sizes of input vectors
outvec=uint8(zeros(Nv*vbytes,1)); % Set output size

if ~IsBigEndian  % Little Endian: typecast, reshape to column-wise, flip, reshape to vector
    cvec = reshape(flipud(reshape(typecast(vec(:),'uint8'),vbytes,Nv)),Nv*vbytes,1);
else   % Big Endian: typecast
    cvec = typecast(vec(:),'uint8');
end

% (:) selector retains size of "outvec"
outvec(:) = cvec;

== matlab function UDP Variable Select/UDP_Pack2/udppack ==
  data: vec input double; vbytes parameter double; outvec output uint8; IsBigEndian parameter boolean
function outvec = udppack(vec,vbytes,IsBigEndian)
Nv = length(vec); % get sizes of input vectors
outvec=uint8(zeros(Nv*vbytes,1)); % Set output size

if ~IsBigEndian  % Little Endian: typecast, reshape to column-wise, flip, reshape to vector
    cvec = reshape(flipud(reshape(typecast(vec(:),'uint8'),vbytes,Nv)),Nv*vbytes,1);
else   % Big Endian: typecast
    cvec = typecast(vec(:),'uint8');
end

% (:) selector retains size of "outvec"
outvec(:) = cvec;

== matlab function UDP Variable Select/UDP_Pack3/udppack ==
  data: vec input double; vbytes parameter double; outvec output uint8; IsBigEndian parameter boolean
function outvec = udppack(vec,vbytes,IsBigEndian)
Nv = length(vec); % get sizes of input vectors
outvec=uint8(zeros(Nv*vbytes,1)); % Set output size

if ~IsBigEndian  % Little Endian: typecast, reshape to column-wise, flip, reshape to vector
    cvec = reshape(flipud(reshape(typecast(vec(:),'uint8'),vbytes,Nv)),Nv*vbytes,1);
else   % Big Endian: typecast
    cvec = typecast(vec(:),'uint8');
end

% (:) selector retains size of "outvec"
outvec(:) = cvec;

== matlab function UDP_Pack/udppack ==
  settings: updateMethod=DISCRETE  sampleTime=Timestep
  data: vec input double; vbytes parameter double; outvec output uint8; IsBigEndian parameter boolean
function outvec = udppack(vec,vbytes,IsBigEndian)
Nv = length(vec); % get sizes of input vectors
outvec=uint8(zeros(Nv*vbytes,1)); % Set output size

if ~IsBigEndian  % Little Endian: typecast, reshape to column-wise, flip, reshape to vector
    cvec = reshape(flipud(reshape(typecast(vec(:),'uint8'),vbytes,Nv)),Nv*vbytes,1);
else   % Big Endian: typecast
    cvec = typecast(vec(:),'uint8');
end

% (:) selector retains size of "outvec"
outvec(:) = cvec;
